simulink model "Slip_compensation_model_by_torque"  (R2019b)
settings: Solver=VariableStepAuto  StartTime=0.0  StopTime=35  FixedStep=10  MaxStep=20e-3  RelTol=1e-4  EnableMultiTasking=on
undefined symbols (not defined in the file): c_e, DiscIntNeverNeededParam, KD, linear_cohesion_model_1, linear_cohesion_model_2, linear_cohesion_model_3, M, R_a
libraries: lib_robotinohardware x5, dspstat3 x3, simulink x3
settings Model: EnablePacing=on  Creator=Олег  LastModifiedBy=Олег

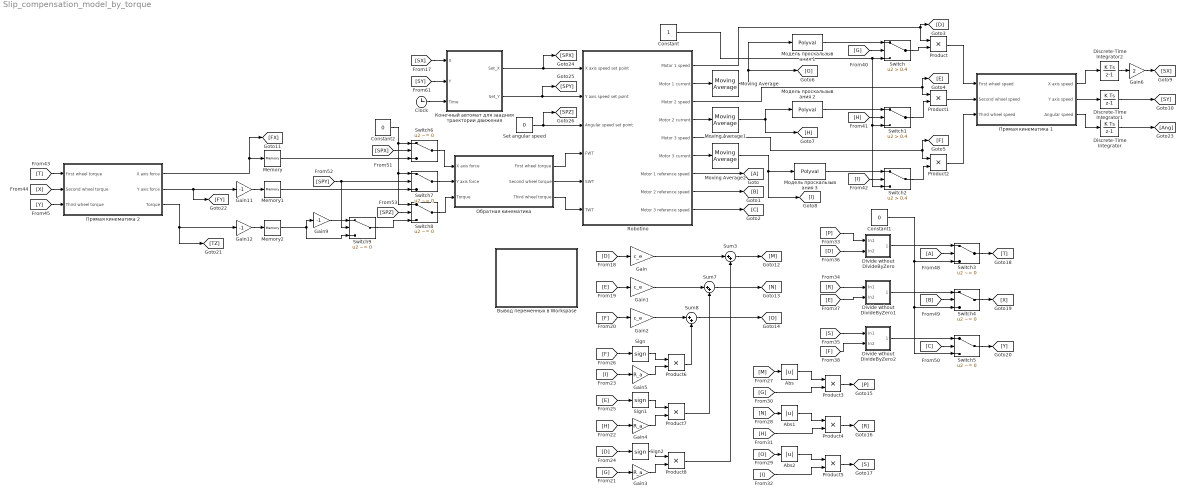
== system Slip_compensation_model_by_torque ==
  Abs : Abs
  Abs1 : Abs
  Abs2 : Abs
  Clock : Clock
  Constant : Constant
  Constant1 : Constant  Value=0
  Constant2 : Constant  Value=0
  Discrete-Time Integrator : DiscreteIntegrator  SampleTime=-1  ICPrevOutput=DiscIntNeverNeededParam  ICPrevScaledInput=DiscIntNeverNeededParam
  Discrete-Time Integrator1 : DiscreteIntegrator  SampleTime=-1  ICPrevOutput=DiscIntNeverNeededParam  ICPrevScaledInput=DiscIntNeverNeededParam
  Discrete-Time Integrator2 : DiscreteIntegrator  SampleTime=-1  ICPrevOutput=DiscIntNeverNeededParam  ICPrevScaledInput=DiscIntNeverNeededParam
  Divide wthout DivideByZero : Subsystem
  Divide wthout DivideByZero1 : Subsystem
  Divide wthout DivideByZero2 : Subsystem
  Gain : Gain  Gain=c_e
  Gain1 : Gain  Gain=c_e
  Gain11 : Gain  Gain=-1
  Gain12 : Gain  Gain=-1
  Gain2 : Gain  Gain=c_e
  Gain3 : Gain  Gain=R_a
  Gain4 : Gain  Gain=R_a
  Gain5 : Gain  Gain=R_a
  Gain6 : Gain  Gain=2
  Gain9 : Gain  Gain=-1
  Memory : Memory
  Memory1 : Memory
  Memory2 : Memory
  Moving Average : dspstat3/Moving Average  Method=Exponential weighting  ForgettingFactorPort=off  SpecifyWindowLength=on  WindowLength=4  ForgettingFactor=0.97  SimulateUsing=Code generation
  Moving Average1 : dspstat3/Moving Average  Method=Exponential weighting  ForgettingFactorPort=off  SpecifyWindowLength=on  WindowLength=4  ForgettingFactor=0.97  SimulateUsing=Code generation
  Moving Average2 : dspstat3/Moving Average  Method=Exponential weighting  ForgettingFactorPort=off  SpecifyWindowLength=on  WindowLength=4  ForgettingFactor=0.97  SimulateUsing=Code generation
  Product{,1..8} (9 alike) : Product
  Robotino : Subsystem
  Set angular speed : Constant  Value=0
  Sign : Signum
  Sign1 : Signum
  Sign2 : Signum
  Sum3 : Sum  Inputs=|++
  Sum7 : Sum  Inputs=|++
  Sum8 : Sum  Inputs=|++
  Switch : Switch  Criteria=u2 > Threshold  Threshold=0.4
  Switch1 : Switch  Criteria=u2 > Threshold  Threshold=0.4
  Switch2 : Switch  Criteria=u2 > Threshold  Threshold=0.4
  Switch{3..9} (7 alike) : Switch  Criteria=u2 ~= 0
  Вывод переменных в Workspase : Subsystem
  Конечный автомат для заадния траектории движения : Stateflow chart  BlockKeywords=__PRM__SERIALIZED__DATA__:Stateflow Chart,Stateflow Diagram  TreatAsAtomicUnit=on
  Модель проскальзывания 1 : Polyval  Coefs=linear_cohesion_model_1
  Модель проскальзывания 2 : Polyval  Coefs=linear_cohesion_model_2
  Модель проскальзывания 3 : Polyval  Coefs=linear_cohesion_model_3
  Обратная кинематика : Subsystem
  Прямая кинематика 1 : Subsystem
  Прямая кинематика 2 : Subsystem
  wires:
  Robotino/9(Motor 3 reference speed) -> [C]
  Robotino/7(Motor 1 reference speed) -> [A]
  Robotino/8(Motor 2 reference speed) -> [B]
  Robotino/1(Motor 1 speed) -> Product/1, [D]
  Robotino/3(Motor 2 speed) -> Product1/1, [E]
  Robotino/5(Motor 3 speed) -> Product2/1, [F]
  Конечный автомат для заадния траектории движения/1(Set_X) -> [SPX], Robotino/1(X axis speed set point)
  Конечный автомат для заадния траектории движения/2(Set_Y) -> [SPY], Robotino/2(Y axis speed set point)
  Product/1 -> Прямая кинематика 1/1("First wheel speed ")
  Product1/1 -> Прямая кинематика 1/2("Second wheel speed ")
  Product2/1 -> Прямая кинематика 1/3("Third wheel speed ")
  Прямая кинематика 1/1(X axis speed) -> Discrete-Time Integrator2/1
  Прямая кинематика 1/2(Y axis speed) -> Discrete-Time Integrator1/1
  Прямая кинематика 1/3(Angular speed) -> Discrete-Time Integrator/1
  Constant/1 -> Switch1/3, Switch2/3, Switch/3
  Модель проскальзывания 1/1 -> Switch/1
  Switch/1 -> Product/2
  Модель проскальзывания 2/1 -> Switch1/1
  Switch1/1 -> Product1/2
  Модель проскальзывания 3/1 -> Switch2/1
  Switch2/1 -> Product2/2
  Robotino/2(Motor 1 current) -> Moving Average/1
  Robotino/4(Motor 2 current) -> Moving Average1/1
  Robotino/6(Motor 3 current) -> Moving Average2/1
  Moving Average/1 -> Модель проскальзывания 1/1, [G]
  Moving Average1/1 -> [H], Модель проскальзывания 2/1
  Moving Average2/1 -> Модель проскальзывания 3/1, [I]
  Gain3/1 -> Product8/2
  Sign2/1 -> Product8/1
  Sign/1 -> Product6/1
  Gain2/1 -> Sum8/1
  Gain5/1 -> Product6/2
  Gain/1 -> Sum3/1
  Gain1/1 -> Sum7/1
  [D] -> Gain/1
  [E] -> Gain1/1
  [F] -> Gain2/1
  Gain4/1 -> Product7/2
  Sign1/1 -> Product7/1
  [G] -> Gain3/1
  [H] -> Gain4/1
  [I] -> Gain5/1
  [D] -> Sign2/1
  [E] -> Sign1/1
  [F] -> Sign/1
  Product6/1 -> Sum8/2
  Product7/1 -> Sum7/2
  Product8/1 -> Sum3/2
  Sum3/1 -> [M]
  Sum7/1 -> [N]
  Sum8/1 -> [O]
  [G] -> Product3/2
  [H] -> Product4/2
  [I] -> Product5/2
  [M] -> Abs/1
  [N] -> Abs1/1
  [O] -> Abs2/1
  Abs/1 -> Product3/1
  Abs1/1 -> Product4/1
  Abs2/1 -> Product5/1
  Product3/1 -> [P]
  Product4/1 -> [R]
  Product5/1 -> [S]
  Discrete-Time Integrator1/1 -> [SY]
  [T] -> Прямая кинематика 2/1("First wheel torque ")
  [X] -> Прямая кинематика 2/2("Second wheel torque ")
  [Y] -> Прямая кинематика 2/3(Third wheel torque)
  Прямая кинематика 2/1(X axis force) -> [FX], Memory/1
  Прямая кинематика 2/3(Torque) -> [TZ], Gain12/1
  Прямая кинематика 2/2(Y axis force) -> [FY], Gain11/1
  [D] -> Divide wthout DivideByZero/2(In2)
  [P] -> Divide wthout DivideByZero/1(In1)
  [E] -> Divide wthout DivideByZero1/2(In2)
  [R] -> Divide wthout DivideByZero1/1(In1)
  [S] -> Divide wthout DivideByZero2/1(In1)
  [F] -> Divide wthout DivideByZero2/2(In2)
  Memory2/1 -> Switch9/3, Gain9/1
  Divide wthout DivideByZero/1(Out1) -> Switch3/1
  Switch3/1 -> [T]
  [A] -> Switch3/2
  Constant1/1 -> Switch3/3, Switch5/3, Switch4/3
  Divide wthout DivideByZero1/1(Out1) -> Switch4/1
  Switch4/1 -> [X]
  [B] -> Switch4/2
  Divide wthout DivideByZero2/1(Out1) -> Switch5/1
  Switch5/1 -> [Y]
  [C] -> Switch5/2
  [SPZ] -> Switch8/2
  Switch6/1 -> Обратная кинематика/1(X axis force)
  Switch7/1 -> Обратная кинематика/2(Y axis force)
  Switch8/1 -> Обратная кинематика/3(Torque)
  Constant2/1 -> Switch8/1, Switch7/1, Switch6/1
  [SPY] -> Switch9/2, Switch7/2
  [SPX] -> Switch6/2
  Обратная кинематика/1(First wheel torque) -> Robotino/4(FWT)
  Обратная кинематика/2(Second wheel torque) -> Robotino/5(SWT)
  Обратная кинематика/3(Third wheel torque) -> Robotino/6(TWT)
  Gain9/1 -> Switch9/1
  Switch9/1 -> Switch8/3
  [SX] -> Конечный автомат для заадния траектории движения/1(X)
  [SY] -> Конечный автомат для заадния траектории движения/2(Y)
  Clock/1 -> Конечный автомат для заадния траектории движения/3(Time)
  Set angular speed/1 -> [SPZ], Robotino/3(Angular speed set point)
  Discrete-Time Integrator2/1 -> Gain6/1
  Gain11/1 -> Memory1/1
  Gain12/1 -> Memory2/1
  [G] -> Switch/2
  [H] -> Switch1/2
  [I] -> Switch2/2
  Memory/1 -> Switch6/3
  Memory1/1 -> Switch7/3
  Discrete-Time Integrator/1 -> [Ang]
  Gain6/1 -> [SX]

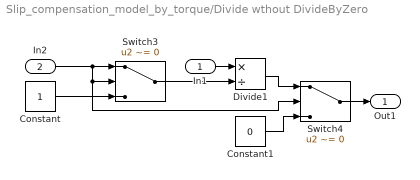
== system Slip_compensation_model_by_torque/Divide wthout DivideByZero ==
  In1 : Inport
  In2 : Inport  Port=2
  Constant : Constant
  Constant1 : Constant  Value=0
  Divide1 : Product  Inputs=*/
  Switch3 : Switch  Criteria=u2 ~= 0
  Switch4 : Switch  Criteria=u2 ~= 0
  Out1 : Outport
  wires:
  Switch3/1 -> Divide1/2
  In1/1 -> Divide1/1
  In2/1 -> Switch3/1, Switch4/2, Switch3/2
  Constant/1 -> Switch3/3
  Divide1/1 -> Switch4/1
  Constant1/1 -> Switch4/3
  Switch4/1 -> Out1/1

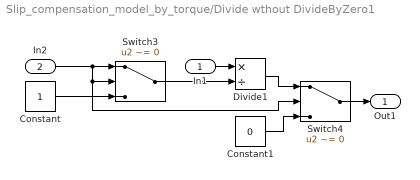
== system Slip_compensation_model_by_torque/Divide wthout DivideByZero1 ==
  In1 : Inport
  In2 : Inport  Port=2
  Constant : Constant
  Constant1 : Constant  Value=0
  Divide1 : Product  Inputs=*/
  Switch3 : Switch  Criteria=u2 ~= 0
  Switch4 : Switch  Criteria=u2 ~= 0
  Out1 : Outport
  wires:
  Switch4/1 -> Out1/1
  Constant1/1 -> Switch4/3
  Divide1/1 -> Switch4/1
  Constant/1 -> Switch3/3
  In1/1 -> Divide1/1
  Switch3/1 -> Divide1/2
  In2/1 -> Switch3/2, Switch4/2, Switch3/1

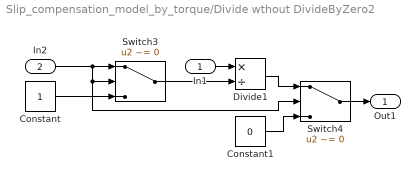
== system Slip_compensation_model_by_torque/Divide wthout DivideByZero2 ==
  In1 : Inport
  In2 : Inport  Port=2
  Constant : Constant
  Constant1 : Constant  Value=0
  Divide1 : Product  Inputs=*/
  Switch3 : Switch  Criteria=u2 ~= 0
  Switch4 : Switch  Criteria=u2 ~= 0
  Out1 : Outport
  wires:
  Switch3/1 -> Divide1/2
  In1/1 -> Divide1/1
  In2/1 -> Switch3/1, Switch4/2, Switch3/2
  Constant/1 -> Switch3/3
  Divide1/1 -> Switch4/1
  Constant1/1 -> Switch4/3
  Switch4/1 -> Out1/1

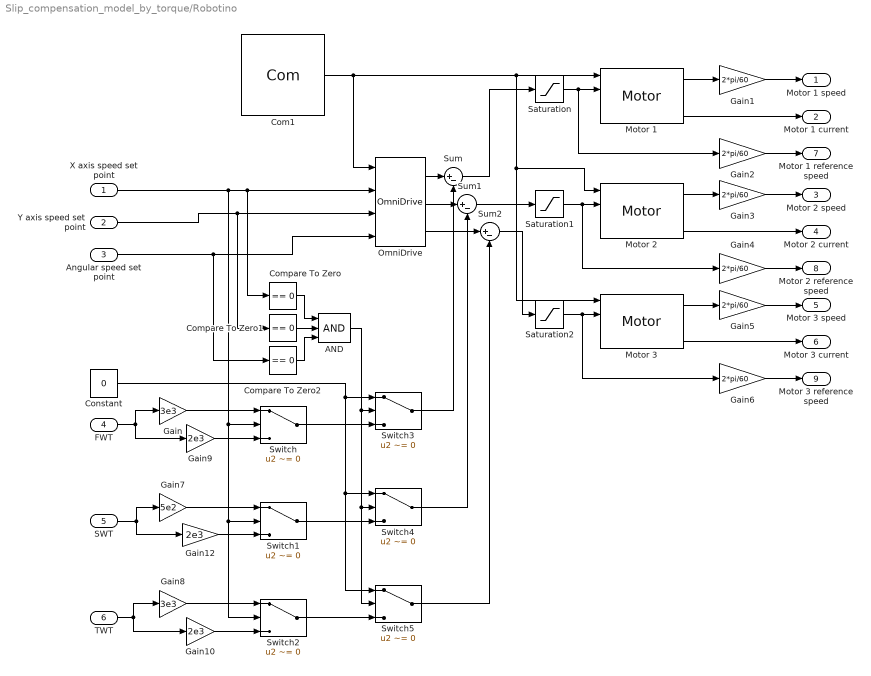
== system Slip_compensation_model_by_torque/Robotino ==
  X axis speed set point : Inport
  Y axis speed set point : Inport  Port=2
  Angular speed set point : Inport  Port=3
  FWT : Inport  Port=4
  SWT : Inport  Port=5
  TWT : Inport  Port=6
  AND : Logic  Inputs=3  IconShape=distinctive  AllPortsSameDT=off  OutDataTypeStr=boolean
  Com1 : lib_robotinohardware/Com  ip='172.26.1.0'
  Compare To Zero : simulink/Logic and Bit Operations/Compare To Zero  relop===  OutDataTypeStr=boolean
  Compare To Zero1 : simulink/Logic and Bit Operations/Compare To Zero  relop===  OutDataTypeStr=boolean
  Compare To Zero2 : simulink/Logic and Bit Operations/Compare To Zero  relop===  OutDataTypeStr=boolean
  Constant : Constant  Value=0
  Gain : Gain  Gain=3e3
  Gain{1..6} (6 alike) : Gain  Gain=2*pi/60
  Gain10 : Gain  Gain=2e3
  Gain12 : Gain  Gain=2e3
  Gain7 : Gain  Gain=5e2
  Gain8 : Gain  Gain=3e3
  Gain9 : Gain  Gain=2e3
  Motor 1 : lib_robotinohardware/Motor  num=0  kp=200  ki=10  kd=0
  Motor 2 : lib_robotinohardware/Motor  num=1  kp=200  ki=10  kd=0
  Motor 3 : lib_robotinohardware/Motor  num=2  kp=200  ki=10  kd=0
  OmniDrive : lib_robotinohardware/OmniDrive
  Saturation : Saturate  UpperLimit=2000  LowerLimit=-2000
  Saturation1 : Saturate  UpperLimit=2000  LowerLimit=-2000
  Saturation2 : Saturate  UpperLimit=2000  LowerLimit=-2000
  Sum : Sum  Inputs=|+-
  Sum1 : Sum  Inputs=|+-
  Sum2 : Sum  Inputs=|+-
  Switch{,1..5} (6 alike) : Switch  Criteria=u2 ~= 0
  Motor 1 speed : Outport
  Motor 1 current : Outport  Port=2
  Motor 2 speed : Outport  Port=3
  Motor 2 current : Outport  Port=4
  Motor 3 speed : Outport  Port=5
  Motor 3 current : Outport  Port=6
  Motor 1 reference speed : Outport  Port=7
  Motor 2 reference speed : Outport  Port=8
  Motor 3 reference speed : Outport  Port=9
  wires:
  Com1/1 -> OmniDrive/1, Motor 1/1, Motor 3/1, Motor 2/1
  Angular speed set point/1 -> Compare To Zero2/1, OmniDrive/4
  Motor 3/3 -> Motor 3 current/1
  Motor 2/1 -> Gain3/1
  Motor 3/1 -> Gain5/1
  Motor 1/1 -> Gain1/1
  Motor 2/3 -> Motor 2 current/1
  X axis speed set point/1 -> OmniDrive/2, Compare To Zero/1, Switch/2, Switch1/2, Switch2/2
  Motor 1/3 -> Motor 1 current/1
  Y axis speed set point/1 -> Compare To Zero1/1, OmniDrive/3
  Gain1/1 -> Motor 1 speed/1
  Gain2/1 -> Motor 1 reference speed/1
  Gain3/1 -> Motor 2 speed/1
  Gain4/1 -> Motor 2 reference speed/1
  Gain5/1 -> Motor 3 speed/1
  Gain6/1 -> Motor 3 reference speed/1
  OmniDrive/1 -> Sum/1
  OmniDrive/2 -> Sum1/1
  OmniDrive/3 -> Sum2/1
  Sum/1 -> Saturation/1
  Sum1/1 -> Saturation1/1
  Sum2/1 -> Saturation2/1
  SWT/1 -> Gain7/1, Gain12/1
  TWT/1 -> Gain10/1, Gain8/1
  Saturation/1 -> Gain2/1, Motor 1/2
  Saturation1/1 -> Gain4/1, Motor 2/2
  Saturation2/1 -> Gain6/1, Motor 3/2
  Gain/1 -> Switch/1
  Gain9/1 -> Switch/3
  FWT/1 -> Gain9/1, Gain/1
  Gain7/1 -> Switch1/1
  Gain12/1 -> Switch1/3
  Gain8/1 -> Switch2/1
  Gain10/1 -> Switch2/3
  Compare To Zero1/1 -> AND/2
  Compare To Zero/1 -> AND/1
  Compare To Zero2/1 -> AND/3
  AND/1 -> Switch5/2, Switch4/2, Switch3/2
  Switch/1 -> Switch3/3
  Constant/1 -> Switch5/1, Switch4/1, Switch3/1
  Switch1/1 -> Switch4/3
  Switch2/1 -> Switch5/3
  Switch3/1 -> Sum/2
  Switch4/1 -> Sum1/2
  Switch5/1 -> Sum2/2

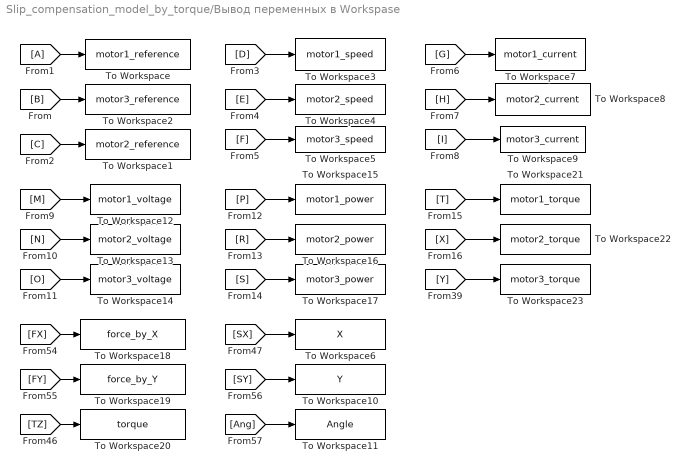
== system Slip_compensation_model_by_torque/Вывод переменных в Workspase ==
  To Workspace : ToWorkspace  VariableName=motor1_reference  SaveFormat=Timeseries  SampleTime=-1
  To Workspace1 : ToWorkspace  VariableName=motor2_reference  SaveFormat=Timeseries  SampleTime=-1
  To Workspace10 : ToWorkspace  VariableName=Y  SaveFormat=Timeseries  SampleTime=-1
  To Workspace11 : ToWorkspace  VariableName=Angle  SaveFormat=Timeseries  SampleTime=-1
  To Workspace12 : ToWorkspace  VariableName=motor1_voltage  SaveFormat=Timeseries  SampleTime=-1
  To Workspace13 : ToWorkspace  VariableName=motor2_voltage  SaveFormat=Timeseries  SampleTime=-1
  To Workspace14 : ToWorkspace  VariableName=motor3_voltage  SaveFormat=Timeseries  SampleTime=-1
  To Workspace15 : ToWorkspace  VariableName=motor1_power  SaveFormat=Timeseries  SampleTime=-1
  To Workspace16 : ToWorkspace  VariableName=motor2_power  SaveFormat=Timeseries  SampleTime=-1
  To Workspace17 : ToWorkspace  VariableName=motor3_power  SaveFormat=Timeseries  SampleTime=-1
  To Workspace18 : ToWorkspace  VariableName=force_by_X  SaveFormat=Timeseries  SampleTime=-1
  To Workspace19 : ToWorkspace  VariableName=force_by_Y  SaveFormat=Timeseries  SampleTime=-1
  To Workspace2 : ToWorkspace  VariableName=motor3_reference  SaveFormat=Timeseries  SampleTime=-1
  To Workspace20 : ToWorkspace  VariableName=torque  SaveFormat=Timeseries  SampleTime=-1
  To Workspace21 : ToWorkspace  VariableName=motor1_torque  SaveFormat=Timeseries  SampleTime=-1
  To Workspace22 : ToWorkspace  VariableName=motor2_torque  SaveFormat=Timeseries  SampleTime=-1
  To Workspace23 : ToWorkspace  VariableName=motor3_torque  SaveFormat=Timeseries  SampleTime=-1
  To Workspace3 : ToWorkspace  VariableName=motor1_speed  SaveFormat=Timeseries  SampleTime=-1
  To Workspace4 : ToWorkspace  VariableName=motor2_speed  SaveFormat=Timeseries  SampleTime=-1
  To Workspace5 : ToWorkspace  VariableName=motor3_speed  SaveFormat=Timeseries  SampleTime=-1
  To Workspace6 : ToWorkspace  VariableName=X  SaveFormat=Timeseries  SampleTime=-1
  To Workspace7 : ToWorkspace  VariableName=motor1_current  SaveFormat=Timeseries  SampleTime=-1
  To Workspace8 : ToWorkspace  VariableName=motor2_current  SaveFormat=Timeseries  SampleTime=-1
  To Workspace9 : ToWorkspace  VariableName=motor3_current  SaveFormat=Timeseries  SampleTime=-1
  wires:
  [B] -> To Workspace2/1
  [A] -> To Workspace/1
  [G] -> To Workspace7/1
  [R] -> To Workspace16/1
  [D] -> To Workspace3/1
  [C] -> To Workspace1/1
  [P] -> To Workspace15/1
  [F] -> To Workspace5/1
  [M] -> To Workspace12/1
  [E] -> To Workspace4/1
  [H] -> To Workspace8/1
  [S] -> To Workspace17/1
  [FY] -> To Workspace19/1
  [I] -> To Workspace9/1
  [TZ] -> To Workspace20/1
  [N] -> To Workspace13/1
  [FX] -> To Workspace18/1
  [SY] -> To Workspace10/1
  [Y] -> To Workspace23/1
  [O] -> To Workspace14/1
  [Ang] -> To Workspace11/1
  [T] -> To Workspace21/1
  [X] -> To Workspace22/1
  [SX] -> To Workspace6/1

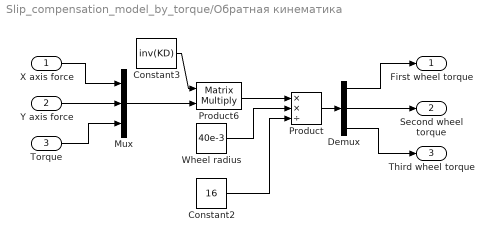
== system Slip_compensation_model_by_torque/Обратная кинематика ==
  X axis force : Inport
  Y axis force : Inport  Port=2
  Torque : Inport  Port=3
  Constant2 : Constant  Value=16
  Constant3 : Constant  Value=inv(KD)
  Demux : Demux  Outputs=3
  Mux : Mux  Inputs=3
  Product : Product  Inputs=**/
  Product6 : Product  Multiplication=Matrix(*)
  Wheel radius : Constant  Value=40e-3
  First wheel torque : Outport
  Second wheel torque : Outport  Port=2
  Third wheel torque : Outport  Port=3
  wires:
  Demux/3 -> Third wheel torque/1
  Demux/2 -> Second wheel torque/1
  Demux/1 -> First wheel torque/1
  Mux/1 -> Product6/2
  Torque/1 -> Mux/3
  X axis force/1 -> Mux/1
  Y axis force/1 -> Mux/2
  Constant3/1 -> Product6/1
  Product6/1 -> Product/1
  Wheel radius/1 -> Product/2
  Constant2/1 -> Product/3
  Product/1 -> Demux/1

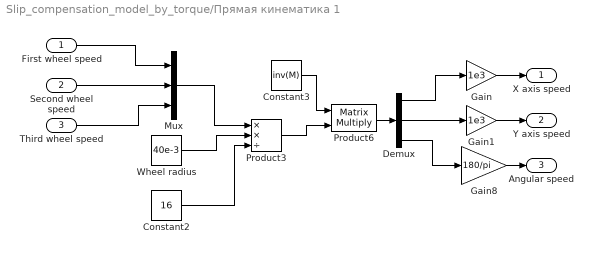
== system Slip_compensation_model_by_torque/Прямая кинематика 1 ==
  "First wheel speed " : Inport
  "Second wheel speed " : Inport  Port=2
  "Third wheel speed " : Inport  Port=3
  Constant2 : Constant  Value=16
  Constant3 : Constant  Value=inv(M)
  Demux : Demux  Outputs=3
  Gain : Gain  Gain=1e3
  Gain1 : Gain  Gain=1e3
  Gain8 : Gain  Gain=180/pi
  Mux : Mux  Inputs=3
  Product3 : Product  Inputs=**/
  Product6 : Product  Multiplication=Matrix(*)
  Wheel radius : Constant  Value=40e-3
  X axis speed : Outport
  Y axis speed : Outport  Port=2
  Angular speed : Outport  Port=3
  wires:
  Demux/2 -> Gain1/1
  Product6/1 -> Demux/1
  Constant3/1 -> Product6/1
  Demux/1 -> Gain/1
  Demux/3 -> Gain8/1
  "Second wheel speed "/1 -> Mux/2
  "First wheel speed "/1 -> Mux/1
  "Third wheel speed "/1 -> Mux/3
  Mux/1 -> Product3/1
  Product3/1 -> Product6/2
  Wheel radius/1 -> Product3/2
  Constant2/1 -> Product3/3
  Gain/1 -> X axis speed/1
  Gain1/1 -> Y axis speed/1
  Gain8/1 -> Angular speed/1

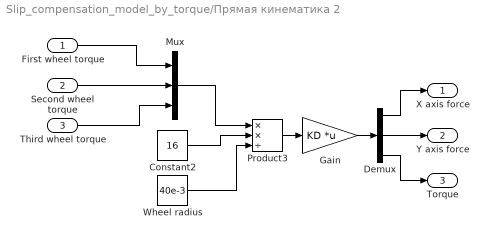
== system Slip_compensation_model_by_torque/Прямая кинематика 2 ==
  "First wheel torque " : Inport
  "Second wheel torque " : Inport  Port=2
  Third wheel torque : Inport  Port=3
  Constant2 : Constant  Value=16
  Demux : Demux  Outputs=3
  Gain : Gain  Gain=KD  Multiplication=Matrix(K*u) (u vector)
  Mux : Mux  Inputs=3
  Product3 : Product  Inputs=**/
  Wheel radius : Constant  Value=40e-3
  X axis force : Outport
  Y axis force : Outport  Port=2
  Torque : Outport  Port=3
  wires:
  Demux/3 -> Torque/1
  Demux/2 -> Y axis force/1
  Demux/1 -> X axis force/1
  Mux/1 -> Product3/1
  Third wheel torque/1 -> Mux/3
  "First wheel torque "/1 -> Mux/1
  "Second wheel torque "/1 -> Mux/2
  Constant2/1 -> Product3/2
  Wheel radius/1 -> Product3/3
  Product3/1 -> Gain/1
  Gain/1 -> Demux/1

== stateflow chart Slip_compensation_model_by_torque/Конечный автомат для заадния траектории движения ==
  state Forward
    during:
    Set_X = 200;
    Set_Y = 0;
  state Stop
    during:
    Set_X = 0;
    Set_Y = 0;
  state Right
    during:
    Set_X = 0;
    Set_Y = 200;
  state Stop1
    entry:
    stop_time = Time;
    during:
    Set_X = 0;
    Set_Y = 0;
  state Stop3
    entry:
    stop_time = Time;
    during:
    Set_X = 0;
    Set_Y = 0;
  state Stop2
    entry:
    stop_time = Time;
    during:
    Set_X = 0;
    Set_Y = 0;
  state Left
    during:
    Set_X = 0;
    Set_Y = -200;
  state Backward
    during:
    Set_X = -200;
    Set_Y = 0
  (default) -> Forward
  Right -> Stop : [Y >= 0]
  Forward -> Stop1 : [X>=900]
  Stop3 -> Right : [(Time - stop_time) > 0.2]
  Stop1 -> Left : [(Time - stop_time) > 0.2]
  Backward -> Stop3 : [X <= 0]
  Left -> Stop2 : [Y <= -400]
  Stop2 -> Backward : [(Time - stop_time) > 0.2]
  data: X input; Y input; Set_X output; Set_Y output; Time input; stop_time local
